simulink model "kinematics_model"  (R2019b)
settings: Solver=VariableStepAuto  StartTime=0.0  StopTime=10.0  RelTol=1e-3
settings Model: Creator=Jamie  LastModifiedBy=Jamie

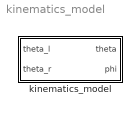
== system kinematics_model ==
  kinematics_model : Subsystem

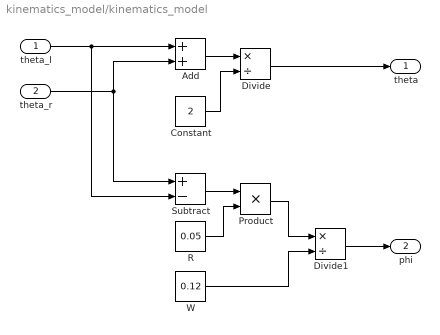
== system kinematics_model/kinematics_model ==
  theta_l : Inport
  theta_r : Inport  Port=2
  Add : Sum
  Constant : Constant  Value=2
  Divide : Product  Inputs=*/
  Divide1 : Product  Inputs=*/
  Product : Product
  R : Constant  Value=0.05
  Subtract : Sum  Inputs=+-
  W : Constant  Value=0.12
  theta : Outport
  phi : Outport  Port=2
  wires:
  theta_l/1 -> Subtract/2, Add/1
  theta_r/1 -> Subtract/1, Add/2
  Add/1 -> Divide/1
  Constant/1 -> Divide/2
  Divide/1 -> theta/1
  Subtract/1 -> Product/1
  R/1 -> Product/2
  Product/1 -> Divide1/1
  W/1 -> Divide1/2
  Divide1/1 -> phi/1
